simulink model "sampleModel1774"  (R2023a)
settings: Solver=VariableStepAuto  StartTime=0.0  StopTime=10.0  RelTol=1e-3
libraries: hdlsllib x6, simulink x1
settings Model: Creator=user1  LastModifiedBy=user1

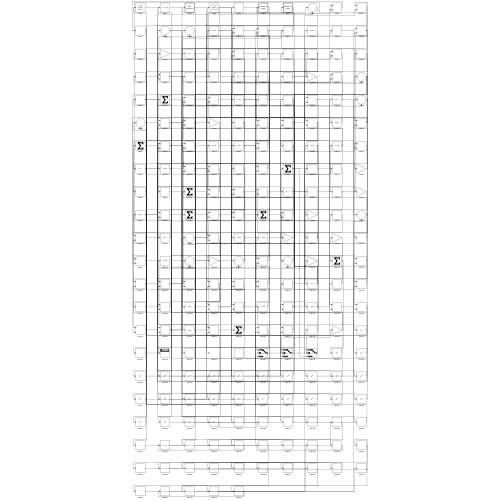
[thumbnail: Simulink's stored preview of the top-level diagram]
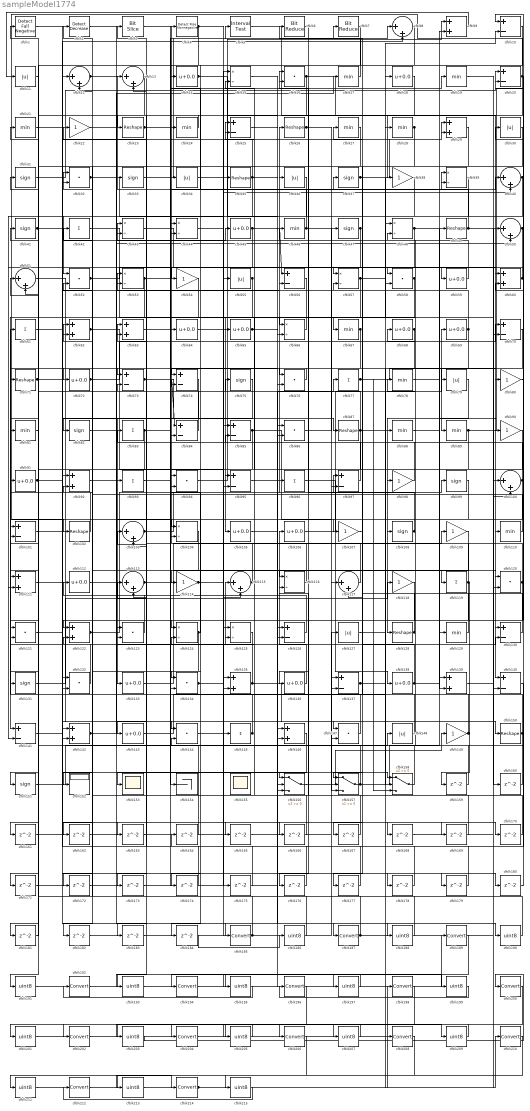
== system sampleModel1774 ==
  cfblk1 : hdlsllib/Logic and Bit Operations/Detect Fall Negative  vinit=0  OutDataTypeStr=boolean
  cfblk{10,20,25,56,70,73..74,84..85,95,97,101,126,130,137,140..141} (17 alike) : Sum  Inputs=+-
  cfblk{8,12..13,40,50..51,100,103,113,115,117} (11 alike) : Sum  Inputs=|++
  cfblk{23,26,35,49,71,87,102,128,150} (9 alike) : Reshape
  cfblk{15,39,43..44,48,53,57,66,104,116,124..125} (12 alike) : Product  Inputs=*/  RndMeth=Zero  SaturateOnIntegerOverflow=on
  cfblk{14,18,45,59,64..65,68..69,72,91,105..106,112,133,136,138,143} (17 alike) : Bias  Bias=0.0  SaturateOnIntegerOverflow=off
  cfblk{22,38,54,80,90,98,107,109,114,118,149} (11 alike) : Gain
  cfblk{31,33,37,41,47,75,82,99,108,131,151} (11 alike) : Signum
  cfblk{11,30,34,36,55,79,127,148} (8 alike) : Abs  SaturateOnIntegerOverflow=off
  cfblk{17,19,21,24,27..28,46,67,78,81,88..89,110,129} (14 alike) : MinMax
  cfblk{9,29,60,62..63,92,111,122,135,139,142,146} (12 alike) : Sum
  cfblk{42,61,77,83,93,96,119,145} (8 alike) : Sum  Inputs=+
  cfblk{16,32,52,58,76,86,94,120..121,123,132,134,144,147} (14 alike) : DotProduct  OutDataTypeStr=Inherit: Inherit via internal rule
  cfblk152 : Display
  cfblk153 : Scope
  cfblk154 : Terminator
  cfblk155 : Scope
      settings: Floating=on
  cfblk156 : Switch  SaturateOnIntegerOverflow=off  InputSameDT=off
  cfblk157 : Switch  SaturateOnIntegerOverflow=off  InputSameDT=off
  cfblk158 : Switch  SaturateOnIntegerOverflow=off  InputSameDT=off
  cfblk{159..184} (26 alike) : Delay  SampleTime=1
  cfblk{185,187,189,192,194,196,198,200,202,204,206,208,210,212,214} (15 alike) : DataTypeConversion  SaturateOnIntegerOverflow=off  RndMeth=Floor
  cfblk{186,188,190..191,193,195,197,199,201,203,205,207,209,211,213,215} (16 alike) : DataTypeConversion  OutDataTypeStr=uint8  SaturateOnIntegerOverflow=off  RndMeth=Floor
  cfblk2 : simulink/Logic and Bit Operations/Detect Decrease  vinit=0.0  OutDataTypeStr=boolean
      settings: LibrarySourceBlock=|
      | hdlsllib/Logic and Bit
      | Operations/Detect
      | Decrease
  cfblk3 : hdlsllib/Logic and Bit Operations/Bit Slice  lidx=7  ridx=0
  cfblk4 : hdlsllib/Logic and Bit Operations/Detect Rise Nonnegative  vinit=0  OutDataTypeStr=boolean
  cfblk5 : hdlsllib/Logic and Bit Operations/Interval Test  IntervalClosedRight=on  uplimit=0.5  IntervalClosedLeft=on  lowlimit=-0.5  OutDataTypeStr=boolean
  cfblk6 : hdlsllib/Logic and Bit Operations/Bit Reduce  mode=AND
  cfblk7 : hdlsllib/Logic and Bit Operations/Bit Reduce  mode=AND
  wires:
  cfblk51/1 -> cfblk147/1
  cfblk96/1 -> cfblk138/1
  cfblk136/1 -> cfblk106/1
  cfblk107/1 -> cfblk43/1
  cfblk20/1 -> cfblk102/1, cfblk123/2, cfblk130/1
  cfblk103/1 -> cfblk99/1, cfblk5/1
  cfblk75/1 -> cfblk133/1
  cfblk116/1 -> cfblk4/1
  cfblk39/1 -> cfblk52/1
  cfblk89/1 -> cfblk10/1, cfblk104/2
  cfblk31/1 -> cfblk20/1
  cfblk135/1 -> cfblk150/1, cfblk115/1
  cfblk133/1 -> cfblk109/1
  cfblk6/1 -> cfblk136/1
  cfblk64/1 -> cfblk105/1
  cfblk35/1 -> cfblk93/1, cfblk25/1, cfblk58/2
  cfblk60/1 -> cfblk54/1, cfblk20/2
  cfblk105/1 -> cfblk77/1
  cfblk100/1 -> cfblk143/1, cfblk43/2
  cfblk26/1 -> cfblk117/1, cfblk176/1
  cfblk55/1 -> cfblk141/1, cfblk74/1
  cfblk68/1 -> cfblk72/1, cfblk158/2
  cfblk92/1 -> cfblk104/1
  cfblk62/1 -> cfblk135/1, cfblk50/2
  cfblk67/1 -> cfblk132/2, cfblk174/1
  cfblk95/1 -> cfblk126/1
  cfblk122/1 -> cfblk26/1, cfblk130/2
  cfblk33/1 -> cfblk8/1
  cfblk43/1 -> cfblk139/1
  cfblk114/1 -> cfblk39/1, cfblk184/1
  cfblk99/1 -> cfblk128/1
  cfblk117/1 -> cfblk63/1
  cfblk79/1 -> cfblk108/1
  cfblk45/1 -> cfblk56/1, cfblk157/2, cfblk74/2
  cfblk106/1 -> cfblk69/1
  cfblk46/1 -> cfblk13/1, cfblk158/1
  cfblk94/1 -> cfblk9/1
  cfblk148/1 -> cfblk27/1
  cfblk36/1 -> cfblk134/1
  cfblk137/1 -> cfblk88/1, cfblk57/2
  cfblk25/1 -> cfblk86/1
  cfblk5/1 -> cfblk140/1
  cfblk145/1 -> cfblk61/1, cfblk52/2
  cfblk59/1 -> cfblk3/1
  cfblk101/1 -> cfblk45/1
  cfblk151/1 -> cfblk148/1
  cfblk47/1 -> cfblk141/2, cfblk116/1
  cfblk24/1 -> cfblk23/1
  cfblk150/1 -> cfblk68/1, cfblk144/2
  cfblk138/1 -> cfblk97/1, cfblk70/1
  cfblk63/1 -> cfblk44/1
  cfblk141/1 -> cfblk56/2
  cfblk84/1 -> cfblk31/1
  cfblk115/1 -> cfblk22/1, cfblk75/1
  cfblk156/1 -> cfblk149/1
  cfblk42/1 -> cfblk139/2
  cfblk97/1 -> cfblk64/1
  cfblk123/1 -> cfblk42/1
  cfblk124/1 -> cfblk94/1, cfblk172/1, cfblk173/1
  cfblk85/1 -> cfblk137/2, cfblk114/1
  cfblk126/1 -> cfblk112/1
  cfblk19/1 -> cfblk140/2
  cfblk70/1 -> cfblk89/1
  cfblk52/1 -> cfblk58/1, cfblk168/1
  cfblk44/1 -> cfblk59/1
  cfblk3/1 -> cfblk34/1
  cfblk37/1 -> cfblk29/1, cfblk70/2
  cfblk71/1 -> cfblk87/1, cfblk163/1
  cfblk13/1 -> cfblk131/1
  cfblk149/1 -> cfblk103/1, cfblk125/2
  cfblk143/1 -> cfblk48/1
  cfblk10/1 -> cfblk94/2
  cfblk108/1 -> cfblk101/1, cfblk16/2
  cfblk72/1 -> cfblk49/1, cfblk12/2
  cfblk73/1 -> cfblk84/1, cfblk125/1
  cfblk147/1 -> cfblk62/1
  cfblk21/1 -> cfblk156/1
  cfblk18/1 -> cfblk113/2
  cfblk132/1 -> cfblk41/1
  cfblk77/1 -> cfblk80/1, cfblk158/3
  cfblk110/1 -> cfblk32/1
  cfblk88/1 -> cfblk90/1
  cfblk120/1 -> cfblk63/2, cfblk157/1
  cfblk78/1 -> cfblk9/2
  cfblk14/1 -> cfblk126/2, cfblk46/1
  cfblk157/1 -> cfblk129/1, cfblk92/2
  cfblk4/1 -> cfblk32/2, cfblk120/1, cfblk40/2
  cfblk130/1 -> cfblk37/1
  cfblk66/1 -> cfblk65/1
  cfblk58/1 -> cfblk97/2, cfblk167/1
  cfblk50/1 -> cfblk110/1, cfblk181/1
  cfblk48/1 -> cfblk60/1, cfblk107/1
  cfblk9/1 -> cfblk11/1
  cfblk41/1 -> cfblk8/2, cfblk144/1
  cfblk2/1 -> cfblk187/1
  cfblk30/1 -> cfblk82/1
  cfblk131/1 -> cfblk118/1
  cfblk29/1 -> cfblk67/1
  cfblk109/1 -> cfblk122/1
  cfblk125/1 -> cfblk122/2
  cfblk16/1 -> cfblk38/1, cfblk73/1
  cfblk69/1 -> cfblk36/1, cfblk15/2, cfblk177/1
  cfblk127/1 -> cfblk79/1
  cfblk104/1 -> cfblk152/1
  cfblk54/1 -> cfblk81/1
  cfblk76/1 -> cfblk71/1
  cfblk32/1 -> cfblk145/1, cfblk169/1
  cfblk22/1 -> cfblk29/2
  cfblk119/1 -> cfblk123/1, cfblk85/2, cfblk159/1
  cfblk61/1 -> cfblk92/1
  cfblk102/1 -> cfblk21/1
  cfblk93/1 -> cfblk19/1
  cfblk38/1 -> cfblk117/2
  cfblk56/1 -> cfblk95/1
  cfblk121/1 -> cfblk24/1
  cfblk1/1 -> cfblk185/1
  cfblk90/1 -> cfblk98/1
  cfblk57/1 -> cfblk28/1, cfblk66/2, cfblk7/1
  cfblk12/1 -> cfblk178/1, cfblk179/1
  cfblk158/1 -> cfblk101/2
  cfblk91/1 -> cfblk12/1, cfblk180/1
  cfblk49/1 -> cfblk100/1, cfblk14/1
  cfblk129/1 -> cfblk78/1
  cfblk53/1 -> cfblk121/1, cfblk40/1
  cfblk86/1 -> cfblk47/1
  cfblk27/1 -> cfblk76/1
  cfblk23/1 -> cfblk76/2, cfblk183/1
  cfblk98/1 -> cfblk16/1
  cfblk11/1 -> cfblk111/1
  cfblk113/1 -> cfblk154/1, cfblk119/1
  cfblk128/1 -> cfblk53/1, cfblk83/1, cfblk44/2
  cfblk40/1 -> cfblk95/2, cfblk111/2, cfblk57/1, cfblk153/1
  cfblk7/1 -> cfblk124/1
  cfblk83/1 -> cfblk151/1, cfblk157/3
  cfblk80/1 -> cfblk30/1
  cfblk34/1 -> cfblk55/1
  cfblk134/1 -> cfblk35/1, cfblk115/2
  cfblk87/1 -> cfblk13/2, cfblk10/2, cfblk39/2, cfblk182/1
  cfblk65/1 -> cfblk96/1, cfblk170/1
  cfblk142/1 -> cfblk17/1, cfblk124/2
  cfblk17/1 -> cfblk6/1
  cfblk112/1 -> cfblk33/1
  cfblk28/1 -> cfblk66/1, cfblk171/1
  cfblk118/1 -> cfblk142/2
  cfblk159/1 -> cfblk48/2
  cfblk139/1 -> cfblk160/1
  cfblk160/1 -> cfblk51/1
  cfblk8/1 -> cfblk161/1
  cfblk161/1 -> cfblk147/2
  cfblk74/1 -> cfblk162/1
  cfblk163/1 -> cfblk135/2
  cfblk140/1 -> cfblk164/1
  cfblk164/1 -> cfblk113/1
  cfblk82/1 -> cfblk165/1
  cfblk165/1 -> cfblk137/1
  cfblk111/1 -> cfblk166/1
  cfblk166/1 -> cfblk62/2
  cfblk167/1 -> cfblk25/2
  cfblk168/1 -> cfblk100/2
  cfblk169/1 -> cfblk53/2
  cfblk170/1 -> cfblk116/2
  cfblk171/1 -> cfblk86/2
  cfblk172/1 -> cfblk84/2
  cfblk173/1 -> cfblk134/2
  cfblk174/1 -> cfblk142/1
  cfblk144/1 -> cfblk175/1
  cfblk175/1 -> cfblk132/1
  cfblk176/1 -> cfblk156/2
  cfblk177/1 -> cfblk103/2
  cfblk178/1 -> cfblk15/1
  cfblk179/1 -> cfblk73/2
  cfblk180/1 -> cfblk60/2
  cfblk181/1 -> cfblk121/2
  cfblk182/1 -> cfblk85/1
  cfblk183/1 -> cfblk156/3
  cfblk185/1 -> cfblk127/1, cfblk51/2
  cfblk184/1 -> cfblk186/1
  cfblk186/1 -> cfblk1/1
  cfblk187/1 -> cfblk50/1, cfblk91/1
  cfblk15/1 -> cfblk188/1
  cfblk188/1 -> cfblk2/1
  cfblk162/1 -> cfblk190/1
  cfblk190/1 -> cfblk146/1
  cfblk81/1 -> cfblk191/1
  cfblk191/1 -> cfblk146/2
  cfblk146/1 -> cfblk193/1
  cfblk193/1 -> cfblk189/1
  cfblk189/1 -> cfblk195/1
  cfblk195/1 -> cfblk192/1
  cfblk192/1 -> cfblk197/1
  cfblk197/1 -> cfblk194/1
  cfblk194/1 -> cfblk199/1
  cfblk199/1 -> cfblk196/1
  cfblk196/1 -> cfblk201/1
  cfblk201/1 -> cfblk198/1
  cfblk198/1 -> cfblk203/1
  cfblk203/1 -> cfblk200/1
  cfblk200/1 -> cfblk205/1
  cfblk205/1 -> cfblk202/1
  cfblk202/1 -> cfblk207/1
  cfblk207/1 -> cfblk204/1
  cfblk204/1 -> cfblk209/1
  cfblk209/1 -> cfblk206/1
  cfblk206/1 -> cfblk211/1
  cfblk211/1 -> cfblk208/1
  cfblk212/1 -> cfblk214/1
  cfblk208/1 -> cfblk213/1
  cfblk213/1 -> cfblk210/1
  cfblk214/1 -> cfblk120/2, cfblk18/1
  cfblk210/1 -> cfblk215/1
  cfblk215/1 -> cfblk212/1
